simulink model "Pointmass_eom_v1_0_R2018B"  (R2018b)
settings: Solver=ode4  StartTime=0.0  StopTime=simInit.TSIM  FixedStep=simInit.dt  MaxStep=simInit.dt  RelTol=1e-3
InitFcn:
  | close all
undefined symbols (not defined in the file or in its folder): base_windspeed, constr, DE2019, DiscIntNeverNeededParam, ENVMT, Lbooth, loiterStates, params, simInit, T
libraries: simulink x26, simulink_extras x2, aerolibconvert2 x1, aerolibwind2 x1
(part 1 of 4)
Description:
  | % Copyright 2020 Delft University of Technology
  | %
  | % Licensed under the Apache License, Version 2.0 (the "License");
  | % you may not use this file except in compliance with the License.
  | % You may obtain a copy of the License at
  | %
  | %      http://www.apache.org/licenses/LICENSE-2.0
  | %
  | % Unless required by applicable law or agreed to in writing, software
  | % distributed under the License is distributed on an "AS IS" BASIS,
  | % WITHOUT WARRANTIES OR CONDITIONS OF ANY KIND, either express or implied.
  | % See the License for the specific language governing permissions and
  | % limitations under the License.
settings Model: SimulationMode=accelerator  ExtModeTrigDuration=100  Creator=Sebastian  LastModifiedBy=dylaneijkelhof
settings SolverCC: SolverJacobianMethodControl=FullAnalytical
settings DataIOCC: SaveFormat=Structure  SignalLogging=off  DSMLogging=off  SaveTime=off  StateSaveName=tmp_raccel_xout  SignalLoggingName=logged_signals  LoggingFileName=log
settings OptimizationCC: EfficientMapNaN2IntZero=off  LifeSpan=inf
settings DebuggingCC: ArtificialAlgebraicLoopMsg=none  SaveWithDisabledLinksMsg=none  SaveWithParameterizedLinksMsg=none  MaskedZcDiagnostic=none  IgnoredZcDiagnostic=none  InheritedTsInSrcMsg=none  TasksWithSamePriorityMsg=none  SigSpecEnsureSampleTimeMsg=none  ParameterPrecisionLossMsg=none  UnconnectedInputMsg=none  UnconnectedOutputMsg=none  UnconnectedLineMsg=none  BusObjectLabelMismatch=none  RootOutportRequireBusObject=none  UnknownTsInhSupMsg=none  ModelReferenceDataLoggingMessage=none  ModelReferenceSymbolNameMessage=none  InitInArrayFormatMsg=none  SFUnusedDataAndEventsDiag=none  SFUnexpectedBacktrackingDiag=none  SFInvalidInputDataAccessInChartInitDiag=none  SFNoUnconditionalDefaultTransitionDiag=none  SFTransitionOutsideNaturalParentDiag=none  SFUnreachableExecutionPathDiag=none  SFUndirectedBroadcastEventsDiag=none  SFTransitionActionBeforeConditionDiag=none  SFTemporalDelaySmallerThanSampleTimeDiag=none  SFSelfTransitionDiag=none  SFExecutionAtInitializationDiag=none  SFMachineParentedDataDiag=none  UnitsInconsistencyMsg=none
settings HardwareCC: TargetBitPerLong=64  TargetBitPerPointer=64  TargetBitPerSizeT=64  TargetBitPerPtrDiffT=64  TargetLongLongMode=on  TargetIntDivRoundTo=Zero  TargetEndianess=LittleEndian  TargetWordSize=64  TargetHWDeviceType=MATLAB Host  ProdEqTarget=off
settings ModelReferenceCC: PropagateSignalLabelsOutOfModel=off
settings SFSimCC: SimUseLocalCustomCode=off
settings CodeAppCC: MaxIdLength=128
settings GRTTargetCC: TargetLangStandard=C89/C90 (ANSI)  CombineOutputUpdateFcns=off  GRTInterface=on
settings ConfigComp: CovMetricSettings=dw  CovHtmlReporting=on  CovSaveCumulativeToWorkspaceVar=on  CovSaveSingleToWorkspaceVar=on  CovExternalEMLEnable=off
settings SimscapeCC: SimscapeNormalizeSystem=off
settings ConfigurationSet: Description=SimMechanics 2G

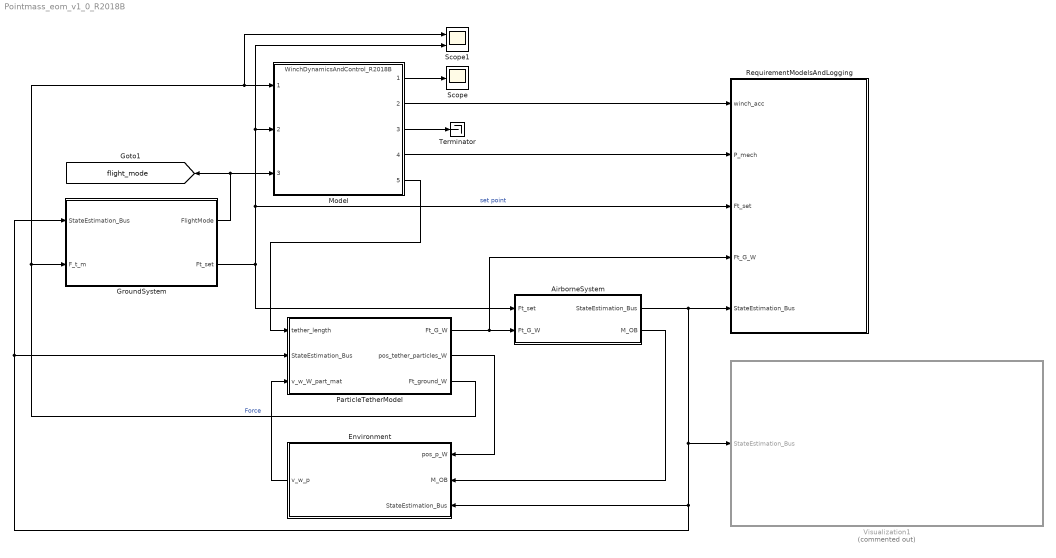
== system Pointmass_eom_v1_0_R2018B ==
  AirborneSystem : Subsystem
  Environment : Subsystem
  GroundSystem : Subsystem
  Model : ModelReference  ModelNameDialog=WinchDynamicsAndControl_R2018B.slx  ModelReferenceVersion=1.22542
  ParticleTetherModel : Subsystem
  RequirementModelsAndLogging : Subsystem  mask{log_sample_time=0.2}
  Scope : Scope
  Scope1 : Scope  NumInputPorts=2
  Terminator : Terminator
  Visualization1 : Subsystem  Commented=on  mask{sample_time_vis=1}
      mask prompts: sample_time_vis "sampletime"
      mask Display: image('DE2019_Aircraft.jpeg')
  tag scope: flight_mode=global
  wires:
  GroundSystem/1(FlightMode) -> Model/3, [flight_mode]
  GroundSystem/2(Ft_set) -> Scope1/2, Model/2, RequirementModelsAndLogging/3(Ft_set), AirborneSystem/1(Ft_set)  "set point"
  AirborneSystem/2(M_OB) -> Environment/2(M_OB)
  ParticleTetherModel/1(Ft_G_W) -> AirborneSystem/2(Ft_G_W), RequirementModelsAndLogging/4(Ft_G_W)
  AirborneSystem/1(StateEstimation_Bus) -> GroundSystem/1(StateEstimation_Bus), ParticleTetherModel/2(StateEstimation_Bus), Environment/3(StateEstimation_Bus), Visualization1/1(StateEstimation_Bus), RequirementModelsAndLogging/5(StateEstimation_Bus)
  ParticleTetherModel/2(pos_tether_particles_W) -> Environment/1(pos_p_W)
  Environment/1(v_w_p) -> ParticleTetherModel/3(v_w_W_part_mat)
  Model/1 -> Scope/1
  ParticleTetherModel/3(Ft_ground_W) -> Scope1/1, Model/1, GroundSystem/2(F_t_m)  "Force"
  Model/3 -> Terminator/1
  Model/2 -> RequirementModelsAndLogging/1(winch_acc)
  Model/4 -> RequirementModelsAndLogging/2(P_mech)
  Model/5 -> ParticleTetherModel/1(tether_length)

== system Pointmass_eom_v1_0_R2018B/AirborneSystem ==
  Ft_set : Inport
  Ft_G_W : Inport  Port=2
  AeroAndPropForces1 : Subsystem
  AttitudeDynamics : Subsystem
  Bus Selector : BusSelector  OutputSignals=airdata
  Delay2 : Delay  DelayLength=1  InitialCondition=[0;0;DE2019.mass*ENVMT.g]
  Dot Product : DotProduct  InputSameDT=on  OutDataTypeStr=Inherit: Inherit via internal rule
  FlightControlSystem : Subsystem
  PointMassEOM : Subsystem
  Sqrt : Sqrt  SaturateOnIntegerOverflow=on
  alpha : Scope  NumInputPorts=2
  mu : Scope  NumInputPorts=2
  StateEstimation_Bus : Outport  VectorParamsAs1DForOutWhenUnconnected=off
  M_OB : Outport  Port=2  VectorParamsAs1DForOutWhenUnconnected=off
  wires:
  PointMassEOM/2(StateEstimation_Bus) -> StateEstimation_Bus/1, FlightControlSystem/4(StateEstimation_Bus), Bus Selector/1  "StateEstimation_Bus"
  PointMassEOM/1(M_OB) -> M_OB/1
  Ft_G_W/1 -> PointMassEOM/1(F_t_W), Dot Product/1, Dot Product/2
  Dot Product/1 -> Sqrt/1
  Ft_set/1 -> FlightControlSystem/1(Ft_set)  "Ft_set"
  Sqrt/1 -> FlightControlSystem/2(Ft_tot)  "Ft_tot"
  FlightControlSystem/3(beta_c) -> PointMassEOM/4(beta_c)
  Delay2/1 -> FlightControlSystem/3(F_a_B_hat)
  AeroAndPropForces1/2(F_a_B) -> Delay2/1, PointMassEOM/6(F_a_B)  "Aero"
  FlightControlSystem/4(throttle) -> AeroAndPropForces1/1(throttle)  "throttle"
  Bus Selector/1 -> AeroAndPropForces1/2(air_data)  "<airdata>"
  AeroAndPropForces1/1(F_p_B) -> PointMassEOM/5(F_p_B)  "Propulsion"
  FlightControlSystem/1(mu_a_cmd) -> mu/1, AttitudeDynamics/1(mu_a_cmd)
  FlightControlSystem/2(alpha_a_cmd) -> alpha/1, AttitudeDynamics/2(alpha_a_cmd)
  AttitudeDynamics/1(mu_a) -> mu/2, PointMassEOM/2(mu_a_c)
  AttitudeDynamics/2(alpha_a) -> PointMassEOM/3(alpha_c), alpha/2

== system Pointmass_eom_v1_0_R2018B/Environment ==
  pos_p_W : Inport
  M_OB : Inport  Port=2
  StateEstimation_Bus : Inport  Port=3
  Bus Selector : BusSelector  OutputSignals=pos_G_O_m
  Constant4 : Constant  Value=ENVMT.windDirection_rad
  Delay : Delay  DelayLength=1  InitialCondition=zeros(3,1)
  Gain : Gain  Gain=-1
  Gain1 : Gain  Gain=-1
  MATLAB Function : MATLAB Function  TreatAsAtomicUnit=on
  Product : Product  Multiplication=Matrix(*)
  Reshape1 : Reshape  OutputDimensionality=Column vector (2-D)
  Selector : Selector  InputPortWidth=3  IndexOptions=Index vector (dialog)  Indices=3  OutputSizes=1
  Selector3 : Selector  InputPortWidth=3*T.np  IndexOptions=Index vector (dialog)  Indices=3:3:3*T.np  OutputSizes=1
  ShearWind : Subsystem  mask{Wdeg=ENVMT.windDirection_rad*180/pi}
      mask prompts: Wdeg "Windirection"
  Windshear : Subsystem
  v_w_p : Outport  VectorParamsAs1DForOutWhenUnconnected=off
  tag scope: vel_W_W=global
  wires:
  Bus Selector/1 -> Selector/1  "<pos_G_O_m>"
  Selector/1 -> Gain/1
  MATLAB Function/1(vec_W) -> Reshape1/1
  StateEstimation_Bus/1 -> Bus Selector/1
  Product/1 -> MATLAB Function/1(vec_O)
  M_OB/1 -> Product/1, Windshear/1(DCM)
  Windshear/1(V_shear_mDs) -> Gain1/1
  Gain1/1 -> Product/2
  Gain/1 -> Windshear/2(altitude)
  Constant4/1 -> MATLAB Function/2(wind_direction_rad)
  Reshape1/1 -> Delay/1
  Selector3/1 -> ShearWind/1(Altitude_p_vec)
  pos_p_W/1 -> Selector3/1
  ShearWind/1(v_w_p) -> v_w_p/1
  Delay/1 -> [vel_W_W]

== system Pointmass_eom_v1_0_R2018B/GroundSystem ==
  StateEstimation_Bus : Inport
  F_t_m : Inport  Port=2
  Bus Selector : BusSelector  OutputSignals=pos_G_W,airdata,longlat
  Demux : Demux  Outputs=2
  GroundControl : Subsystem
  Selector : Selector  InputPortWidth=3  IndexOptions=Index vector (dialog)  Indices=1  OutputSizes=1
  Selector1 : Selector  InputPortWidth=3  IndexOptions=Index vector (dialog)  Indices=1  OutputSizes=1
  Selector3 : Selector  InputPortWidth=2  IndexOptions=Index vector (dialog)  Indices=1  OutputSizes=1
  StateMachine : Subsystem
  FlightMode : Outport  VectorParamsAs1DForOutWhenUnconnected=off
  Ft_set : Outport  Port=2  VectorParamsAs1DForOutWhenUnconnected=off
  tag scope: phi0_update=global
  wires:
  Selector/1 -> StateMachine/2(Va)
  Bus Selector/2 -> Selector/1  "<airdata>"
  Bus Selector/1 -> StateMachine/1(pos_W)  "<pos_G_W>"
  StateEstimation_Bus/1 -> Bus Selector/1
  Demux/1 -> StateMachine/3(longitude)
  StateMachine/2(Ft_set) -> Ft_set/1
  Demux/2 -> StateMachine/4(lattitude)
  [cross_track_error] -> StateMachine/6(cross_track_error)
  F_t_m/1 -> StateMachine/7(F_t_m)
  Bus Selector/3 -> Selector3/1, Demux/1  "<longlat>"
  StateMachine/1(FlightMode) -> GroundControl/1(flightMode), FlightMode/1
  Selector1/1 -> [phi0_update]
  GroundControl/1(path_update) -> Selector1/1, StateMachine/5(path_update)
  Selector3/1 -> GroundControl/2(long)
  GroundControl/2(lat_init) -> StateMachine/8(lat_init)

== system Pointmass_eom_v1_0_R2018B/ParticleTetherModel ==
  tether_length : Inport
  StateEstimation_Bus : Inport  Port=2
  v_w_W_part_mat : Inport  Port=3
  Bus Selector : BusSelector  OutputSignals=pos_G_W,vel_W
  Delay : Delay  DelayLength=1  InitialCondition=zeros(3,1)
  Delay1 : Delay  DelayLength=1  InitialCondition=zeros(3,1)
  Dot Product : DotProduct  InputSameDT=on  OutDataTypeStr=Inherit: Inherit via internal rule
  Dot Product1 : DotProduct  Commented=on  InputSameDT=on  OutDataTypeStr=Inherit: Inherit via internal rule
  Gain : Gain  Gain=-1
  Integrator : Integrator  InitialCondition=simInit.vel_p_init
  Integrator1 : Integrator  InitialCondition=simInit.pos_p_init
  Scope : Scope  Commented=on  NumInputPorts=2
  Selector1 : Selector  InputPortWidth=3*T.np  IndexOptions=Index vector (dialog)  Indices=3:3:3*T.np  OutputSizes=1
  Selector2 : Selector  InputPortWidth=3*T.np  IndexOptions=Index vector (dialog)  Indices=2:3:3*T.np-1  OutputSizes=1
  Selector3 : Selector  InputPortWidth=3*T.np  IndexOptions=Index vector (dialog)  Indices=1:3:3*T.np-2  OutputSizes=1
  Sqrt : Sqrt  SaturateOnIntegerOverflow=on
  Sqrt1 : Sqrt  Commented=on  SaturateOnIntegerOverflow=on
  Tethermodel : ModelReference  ModelNameDialog=Tethermodel_R2018B.slx  ModelReferenceVersion=1.22531
  Ft_G_W : Outport  VectorParamsAs1DForOutWhenUnconnected=off
  pos_tether_particles_W : Outport  Port=2  VectorParamsAs1DForOutWhenUnconnected=off
  Ft_ground_W : Outport  Port=3  VectorParamsAs1DForOutWhenUnconnected=off
  tag scope: p_t_x=global, p_t_y=global, p_t_z=global
  wires:
  Tethermodel/2 -> Delay/1
  Tethermodel/3 -> Gain/1
  Gain/1 -> Delay1/1
  v_w_W_part_mat/1 -> Tethermodel/6
  Integrator/1 -> Integrator1/1, Tethermodel/1
  Tethermodel/1 -> Integrator/1
  Delay/1 -> Dot Product/2, Dot Product/1
  StateEstimation_Bus/1 -> Bus Selector/1
  Bus Selector/1 -> Tethermodel/4  "<pos_G_W>"
  Bus Selector/2 -> Tethermodel/5  "<vel_W>"
  Selector3/1 -> [p_t_x]
  Selector1/1 -> [p_t_z]
  Selector2/1 -> [p_t_y]
  Integrator1/1 -> Tethermodel/2, Selector3/1, Selector2/1, Selector1/1, pos_tether_particles_W/1
  Dot Product/1 -> Sqrt/1
  Sqrt/1 -> Ft_ground_W/1, Scope/1
  Dot Product1/1 -> Sqrt1/1
  Sqrt1/1 -> Scope/2
  Delay1/1 -> Dot Product1/1, Dot Product1/2, Ft_G_W/1
  tether_length/1 -> Tethermodel/3

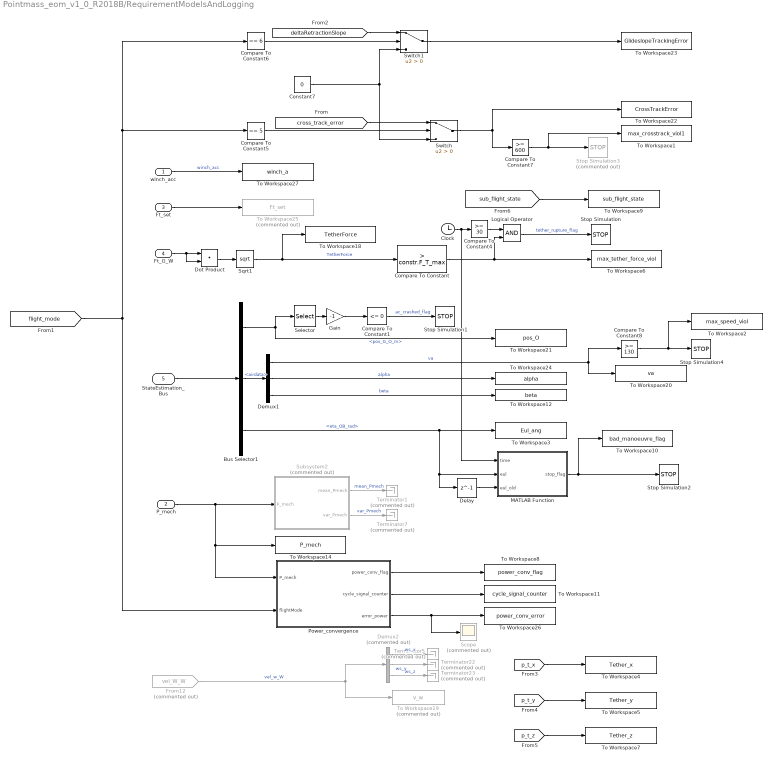
== system Pointmass_eom_v1_0_R2018B/RequirementModelsAndLogging ==
  winch_acc : Inport
  P_mech : Inport  Port=2
  Ft_set : Inport  Port=3
  Ft_G_W : Inport  Port=4
  StateEstimation_Bus : Inport  Port=5
  Bus Selector1 : BusSelector  OutputSignals=pos_G_O_m,airdata,eta_OB_rad
  Clock : Clock
  Compare To Constant : simulink/Logic and Bit Operations/Compare To Constant  relop=>  const=constr.F_T_max  OutDataTypeStr=boolean
  Compare To Constant1 : simulink/Logic and Bit Operations/Compare To Constant  relop=<=  const=0  OutDataTypeStr=boolean
  Compare To Constant4 : simulink/Logic and Bit Operations/Compare To Constant  relop=>=  const=30  OutDataTypeStr=boolean
  Compare To Constant5 : simulink/Logic and Bit Operations/Compare To Constant  relop===  const=5  OutDataTypeStr=boolean
  Compare To Constant6 : simulink/Logic and Bit Operations/Compare To Constant  relop===  const=6  OutDataTypeStr=boolean
  Compare To Constant7 : simulink/Logic and Bit Operations/Compare To Constant  relop=>=  const=600  OutDataTypeStr=boolean
  Compare To Constant8 : simulink/Logic and Bit Operations/Compare To Constant  relop=>=  const=130  OutDataTypeStr=boolean
  Constant7 : Constant  Value=0
  Delay : Delay  DelayLength=1  InitialCondition=zeros(3,1)
  Demux1 : Demux  Outputs=3
  Demux2 : Demux  Commented=on  Outputs=3
  Dot Product : DotProduct  InputSameDT=on  OutDataTypeStr=Inherit: Inherit via internal rule
  From12 : From  Commented=on  GotoTag=vel_W_W  TagVisibility=global
  Gain : Gain  Gain=-1
  Logical Operator : Logic  AllPortsSameDT=off  OutDataTypeStr=boolean
  MATLAB Function : MATLAB Function  TreatAsAtomicUnit=on
  Power_convergence : Subsystem  mask{sample_time=simInit.Ts_power_conv_check, threshold=130000}
  Scope : Scope  Commented=on
  Selector : Selector  InputPortWidth=3  IndexOptions=Index vector (dialog)  Indices=3  OutputSizes=1
  Sqrt1 : Sqrt  SaturateOnIntegerOverflow=on
  Stop Simulation{,1..2,4} (4 alike) : Stop
  Stop Simulation3 : Stop  Commented=on
  Subsystem2 : Subsystem  Commented=on
  Switch : Switch  Criteria=u2 > Threshold
  Switch1 : Switch  Criteria=u2 > Threshold
  Terminator{1,5,7,22..23} (5 alike) : Terminator  Commented=on
  To Workspace1 : ToWorkspace  VariableName=max_crosstrack_viol1  SampleTime=-1
      settings: MaxDataPoints=1
  To Workspace10 : ToWorkspace  VariableName=bad_manoeuvre_flag  SampleTime=-1
      settings: MaxDataPoints=1
  To Workspace11 : ToWorkspace  VariableName=cycle_signal_counter  SaveFormat=Timeseries  SampleTime=-1
      settings: MaxDataPoints=1  Save2DSignal=2-D array (concatenate along first dimension)
  To Workspace12 : ToWorkspace  VariableName=beta  SaveFormat=Timeseries  SampleTime=simInit.AttLoggingTs
      settings: Save2DSignal=2-D array (concatenate along first dimension)
  To Workspace14 : ToWorkspace  VariableName=P_mech  SaveFormat=Timeseries  SampleTime=simInit.PLoggingTs
  To Workspace18 : ToWorkspace  VariableName=TetherForce  SaveFormat=Timeseries  SampleTime=simInit.FtLoggingTs
  To Workspace19 : ToWorkspace  Commented=on  VariableName=v_w  SaveFormat=Timeseries  SampleTime=simInit.vWLoggingTs
  To Workspace2 : ToWorkspace  VariableName=max_speed_viol  SampleTime=-1
      settings: MaxDataPoints=1
  To Workspace20 : ToWorkspace  VariableName=va  SaveFormat=Timeseries  SampleTime=simInit.PLoggingTs
      settings: Save2DSignal=2-D array (concatenate along first dimension)
  To Workspace21 : ToWorkspace  VariableName=pos_O  SaveFormat=Timeseries  SampleTime=simInit.PLoggingTs
      settings: Save2DSignal=2-D array (concatenate along first dimension)
  To Workspace22 : ToWorkspace  VariableName=CrossTrackError  SaveFormat=Timeseries  SampleTime=simInit.CteLoggingTs
      settings: Save2DSignal=2-D array (concatenate along first dimension)
  To Workspace23 : ToWorkspace  VariableName=GlideslopeTrackingError  SaveFormat=Timeseries  SampleTime=simInit.GSLoggingTs
      settings: Save2DSignal=2-D array (concatenate along first dimension)
  To Workspace24 : ToWorkspace  VariableName=alpha  SaveFormat=Timeseries  SampleTime=simInit.AttLoggingTs
      settings: Save2DSignal=2-D array (concatenate along first dimension)
  To Workspace25 : ToWorkspace  Commented=on  VariableName=Ft_set  SaveFormat=Timeseries  SampleTime=simInit.FtLoggingTs
  To Workspace26 : ToWorkspace  VariableName=power_conv_error  SaveFormat=Timeseries  SampleTime=-1
      settings: Save2DSignal=2-D array (concatenate along first dimension)
  To Workspace27 : ToWorkspace  VariableName=winch_a  SaveFormat=Timeseries  SampleTime=simInit.PLoggingTs
  To Workspace3 : ToWorkspace  VariableName=Eul_ang  SaveFormat=Timeseries  SampleTime=simInit.PLoggingTs
      settings: Save2DSignal=2-D array (concatenate along first dimension)
  To Workspace4 : ToWorkspace  VariableName=Tether_x  SaveFormat=Timeseries  SampleTime=simInit.PLoggingTs
      settings: Save2DSignal=2-D array (concatenate along first dimension)
  To Workspace5 : ToWorkspace  VariableName=Tether_y  SaveFormat=Timeseries  SampleTime=simInit.PLoggingTs
      settings: Save2DSignal=2-D array (concatenate along first dimension)
  To Workspace6 : ToWorkspace  VariableName=max_tether_force_viol  SampleTime=-1
      settings: MaxDataPoints=1
  To Workspace7 : ToWorkspace  VariableName=Tether_z  SaveFormat=Timeseries  SampleTime=simInit.PLoggingTs
      settings: Save2DSignal=2-D array (concatenate along first dimension)
  To Workspace8 : ToWorkspace  VariableName=power_conv_flag  SampleTime=-1
      settings: MaxDataPoints=1
  To Workspace9 : ToWorkspace  VariableName=sub_flight_state  SaveFormat=Timeseries  SampleTime=simInit.FtLoggingTs
  wires:
  Bus Selector1/1 -> Selector/1, To Workspace21/1  "<pos_G_O_m>"
  Gain/1 -> Compare To Constant1/1
  Compare To Constant1/1 -> Stop Simulation1/1  "ac_crashed_flag"
  Selector/1 -> Gain/1
  winch_acc/1 -> To Workspace27/1  "winch_acc"
  Logical Operator/1 -> Stop Simulation/1  "tether_rupture_flag"
  Sqrt1/1 -> To Workspace18/1, Compare To Constant/1  "TetherForce"
  StateEstimation_Bus/1 -> Bus Selector1/1
  Power_convergence/1(power_conv_flag) -> To Workspace8/1
  Power_convergence/2(cycle_signal_counter) -> To Workspace11/1
  From12/1 -> Demux2/1, To Workspace19/1  "vel_w_W"
  Bus Selector1/2 -> Demux1/1  "<airdata>"
  Switch/1 -> To Workspace22/1, Compare To Constant7/1
  Subsystem2/1(mean_Pmech) -> Terminator1/1  "mean_Pmech"
  Subsystem2/2(var_Pmech) -> Terminator7/1  "var_Pmech"
  Demux1/1 -> Compare To Constant8/1, To Workspace20/1  "va"
  Demux1/2 -> To Workspace24/1  "alpha"
  Demux1/3 -> To Workspace12/1  "beta"
  Demux2/3 -> Terminator23/1  "ws_z"
  Demux2/2 -> Terminator22/1  "ws_y"
  Demux2/1 -> Terminator5/1  "ws_x"
  Ft_G_W/1 -> Dot Product/2, Dot Product/1
  Dot Product/1 -> Sqrt1/1
  Clock/1 -> MATLAB Function/1(time), Compare To Constant4/1
  Compare To Constant4/1 -> Logical Operator/1
  Compare To Constant/1 -> Logical Operator/2, To Workspace6/1
  [flight_mode] -> Compare To Constant6/1, Compare To Constant5/1, Power_convergence/2(flightMode)
  P_mech/1 -> Power_convergence/1(P_mech), To Workspace14/1, Subsystem2/1(P_mech)
  Compare To Constant5/1 -> Switch/2
  [cross_track_error] -> Switch/1
  Switch1/1 -> To Workspace23/1
  [deltaRetractionSlope] -> Switch1/1
  Compare To Constant6/1 -> Switch1/2
  Constant7/1 -> Switch1/3, Switch/3
  Ft_set/1 -> To Workspace25/1
  Power_convergence/3(error_power) -> Scope/1, To Workspace26/1
  Compare To Constant7/1 -> Stop Simulation3/1, To Workspace1/1
  Compare To Constant8/1 -> To Workspace2/1, Stop Simulation4/1
  [p_t_y] -> To Workspace5/1
  [p_t_x] -> To Workspace4/1
  [p_t_z] -> To Workspace7/1
  [sub_flight_state] -> To Workspace9/1
  Bus Selector1/3 -> To Workspace3/1, Delay/1, MATLAB Function/2(eul)  "<eta_OB_rad>"
  Delay/1 -> MATLAB Function/3(eul_old)
  MATLAB Function/1(stop_flag) -> Stop Simulation2/1, To Workspace10/1

== system Pointmass_eom_v1_0_R2018B/Visualization1 ==
  StateEstimation_Bus : Inport
  Bus Selector : BusSelector  OutputSignals=pos_G_O_m,eta_OB_rad
  Clock2 : Clock
  Constant : Constant  Value=ENVMT.windDirection_rad
  Constant1 : Constant  Value=params.a_booth
  Constant2 : Constant  Value=params.b_booth
  Constant3 : Constant  Value=T.np
  Mux : Mux  Inputs=9
  Mux1 : Mux  Inputs=3
  Rate Transition1 : RateTransition  OutPortSampleTime=sample_time_vis
  Rate Transition2 : RateTransition  InitialCondition=simInit.pos_O_init  OutPortSampleTime=sample_time_vis
  Rate Transition3 : RateTransition  InitialCondition=zeros(3,1)  OutPortSampleTime=sample_time_vis
  Rate Transition4 : RateTransition  OutPortSampleTime=sample_time_vis
  Rate Transition5 : RateTransition  InitialCondition=simInit.pos_p_init(1:3:3*T.np-2)  OutPortSampleTime=sample_time_vis
  Rate Transition6 : RateTransition  OutPortSampleTime=sample_time_vis
  Rate Transition7 : RateTransition  InitialCondition=simInit.pos_p_init(2:3:3*T.np-1)  OutPortSampleTime=sample_time_vis
  Rate Transition8 : RateTransition  InitialCondition=simInit.pos_p_init(3:3:3*T.np)  OutPortSampleTime=sample_time_vis
  Rate Transition9 : RateTransition  InitialCondition=[params.a_booth;params.b_booth;params.phi0_booth]  OutPortSampleTime=sample_time_vis
  To Workspace : ToWorkspace  Commented=on  VariableName=save_visualization  SaveFormat=Timeseries  SampleTime=-1
  advanced_graphical_model : MATLABFcn  MATLABFcn=drawVehicle_v3st_twin  OutputDimensions=0
  wires:
  Bus Selector/2 -> Rate Transition3/1  "<eta_OB_rad>"
  Bus Selector/1 -> Rate Transition2/1  "<pos_G_O_m>"
  StateEstimation_Bus/1 -> Bus Selector/1
  Rate Transition3/1 -> Mux/2
  Rate Transition2/1 -> Mux/1
  Constant3/1 -> Rate Transition6/1
  Rate Transition6/1 -> Mux/4
  Mux/1 -> advanced_graphical_model/1, To Workspace/1  "visualization_stuff"
  Clock2/1 -> Rate Transition1/1
  Rate Transition1/1 -> Mux/3
  Rate Transition4/1 -> Mux/5
  Constant/1 -> Rate Transition4/1
  [p_t_z] -> Rate Transition8/1
  [p_t_y] -> Rate Transition7/1
  [p_t_x] -> Rate Transition5/1
  Rate Transition5/1 -> Mux/7
  Rate Transition7/1 -> Mux/8
  Rate Transition8/1 -> Mux/9
  Mux1/1 -> Rate Transition9/1
  Rate Transition9/1 -> Mux/6
  Constant1/1 -> Mux1/1
  Constant2/1 -> Mux1/2
  [phi0_update] -> Mux1/3

== system Pointmass_eom_v1_0_R2018B/AirborneSystem/AeroAndPropForces1 ==
  throttle : Inport
  air_data : Inport  Port=2
  1-D Lookup Table : Lookup_n-D  NumberOfTableDimensions=1  BreakpointsForDimension1=DE2019.initAircraft.alpha  BreakpointsForDimension2=[1 1]  Table=DE2019.initAircraft.wing_cL_Static'  InternalRulePriority=Speed  RndMeth=Simplest  InputSameDT=on
  1-D Lookup Table1 : Lookup_n-D  NumberOfTableDimensions=1  BreakpointsForDimension1=DE2019.initAircraft.alpha  BreakpointsForDimension2=[1 1]  Table=DE2019.initAircraft.wing_cD_Static'  InternalRulePriority=Speed  RndMeth=Simplest  InputSameDT=on
  1-D Lookup Table2 : Lookup_n-D  NumberOfTableDimensions=1  BreakpointsForDimension1=DE2019.alpha  BreakpointsForDimension2=[1 1]  Table=DE2019.el_cL'  InternalRulePriority=Speed  RndMeth=Simplest  InputSameDT=on
  1-D Lookup Table3 : Lookup_n-D  NumberOfTableDimensions=1  BreakpointsForDimension1=DE2019.alpha  BreakpointsForDimension2=[1 1]  Table=DE2019.el_cD'  InternalRulePriority=Speed  RndMeth=Simplest  InputSameDT=on
  1-D Lookup Table4 : Lookup_n-D  NumberOfTableDimensions=1  BreakpointsForDimension1=DE2019.alpha  BreakpointsForDimension2=[1 1]  Table=DE2019.vs_cL'  InternalRulePriority=Speed  RndMeth=Simplest  InputSameDT=on
  1-D Lookup Table5 : Lookup_n-D  NumberOfTableDimensions=1  BreakpointsForDimension1=DE2019.alpha  BreakpointsForDimension2=[1 1]  Table=DE2019.vs_cD'  InternalRulePriority=Speed  RndMeth=Simplest  InputSameDT=on
  Aero_prop : MATLAB Function  TreatAsAtomicUnit=on
  Radians to Degrees : simulink_extras/Transformations/Radians to Degrees
  Radians to Degrees1 : simulink_extras/Transformations/Radians to Degrees
  Saturation : Saturate  UpperLimit=max(DE2019.initAircraft.alpha)  LowerLimit=min(DE2019.initAircraft.alpha)
  Saturation1 : Saturate  UpperLimit=max(DE2019.alpha)  LowerLimit=min(DE2019.alpha)
  Saturation2 : Saturate  UpperLimit=max(DE2019.alpha)  LowerLimit=min(DE2019.alpha)
  Scope : Scope  Commented=on
  Selector : Selector  Commented=on  InputPortWidth=3  IndexOptions=Index vector (dialog)  Indices=[1]  OutputSizes=1
  Selector1 : Selector  Commented=on  InputPortWidth=3  IndexOptions=Index vector (dialog)  Indices=2  OutputSizes=1
  Selector2 : Selector  Commented=on  InputPortWidth=3  IndexOptions=Index vector (dialog)  Indices=3  OutputSizes=1
  Velocity : Scope  Commented=on
  alpha : Scope  Commented=on
  alpha select : Selector  InputPortWidth=3  IndexOptions=Index vector (dialog)  Indices=2  OutputSizes=1
  beta select : Selector  InputPortWidth=3  IndexOptions=Index vector (dialog)  Indices=3  OutputSizes=1
  F_p_B : Outport  VectorParamsAs1DForOutWhenUnconnected=off
  F_a_B : Outport  Port=2  VectorParamsAs1DForOutWhenUnconnected=off
  wires:
  Aero_prop/1(F_p_B) -> F_p_B/1
  throttle/1 -> Aero_prop/2(delta_t)
  Selector/1 -> Velocity/1
  Selector1/1 -> alpha/1
  1-D Lookup Table/1 -> Aero_prop/3(cl_w)
  1-D Lookup Table1/1 -> Aero_prop/4(cd_w)
  Saturation/1 -> 1-D Lookup Table/1, 1-D Lookup Table1/1
  Saturation1/1 -> 1-D Lookup Table3/1, 1-D Lookup Table2/1
  alpha select/1 -> Radians to Degrees/1
  Radians to Degrees/1 -> Saturation1/1, Saturation/1
  1-D Lookup Table2/1 -> Aero_prop/5(cl_e)
  1-D Lookup Table3/1 -> Aero_prop/6(cd_e)
  1-D Lookup Table4/1 -> Aero_prop/7(cl_r)
  1-D Lookup Table5/1 -> Aero_prop/8(cd_r)
  beta select/1 -> Radians to Degrees1/1
  Radians to Degrees1/1 -> Saturation2/1
  Saturation2/1 -> 1-D Lookup Table4/1, 1-D Lookup Table5/1
  Selector2/1 -> Scope/1
  Aero_prop/2(F_a_B) -> F_a_B/1, Selector2/1
  air_data/1 -> Selector/1, Selector1/1, Aero_prop/1(airdata), beta select/1, alpha select/1

== system Pointmass_eom_v1_0_R2018B/AirborneSystem/AttitudeDynamics ==
  mu_a_cmd : Inport
  alpha_a_cmd : Inport  Port=2
  Scope : Scope  Commented=on  NumInputPorts=2
  SecondOrderReferenceModel_alpha_a : Subsystem  mask{omega0_max=params.w0_alpha, omega0_min=0, dynP_max=1.5312e+03, dynP_min=245.0000, zeta0=0.7, y_max=constr.alpha_a_max, y_min=constr.alpha_a_min, yd_max=inf, yd_min=-inf, y2d_max=inf, y2d_min=-inf}
      mask prompts: dynP_max "max. dynamic pressure"; dynP_min "min. dynamic pressure"
  SecondOrderReferenceModel_mu_a : Subsystem  mask{omega0_max=params.w0_mu, omega0_min=0, dynP_max=1.5312e+03, dynP_min=245.0000, zeta0=1, y_max=constr.mu_a_max, y_min=-constr.mu_a_max, yd_max=inf, yd_min=-inf, y2d_max=inf, y2d_min=-inf}
      mask prompts: dynP_max "max. dynamic pressure"; dynP_min "min. dynamic pressure"
  mu_a : Outport  VectorParamsAs1DForOutWhenUnconnected=off
  alpha_a : Outport  Port=2  VectorParamsAs1DForOutWhenUnconnected=off
  wires:
  mu_a_cmd/1 -> SecondOrderReferenceModel_mu_a/1(y_cmd)
  SecondOrderReferenceModel_alpha_a/1(y_ref) -> Scope/1, alpha_a/1  "alpha_a"
  alpha_a_cmd/1 -> Scope/2, SecondOrderReferenceModel_alpha_a/1(y_cmd)
  SecondOrderReferenceModel_mu_a/1(y_ref) -> mu_a/1  "mu_a"

== system Pointmass_eom_v1_0_R2018B/AirborneSystem/FlightControlSystem ==
  Ft_set : Inport
  Ft_tot : Inport  Port=2
  F_a_B_hat : Inport  Port=3
  StateEstimation_Bus : Inport  Port=4
  AirspeedController : Subsystem
  Bus Selector : BusSelector  OutputSignals=airdata,pathangles_a
  Constant : Constant  Value=0
  PathFollowingController : Subsystem
  Rate Transition : RateTransition  OutPortSampleTime=0.001
  Rate Transition1 : RateTransition  OutPortSampleTime=0.001
  Selector : Selector  InputPortWidth=3  IndexOptions=Index vector (dialog)  Indices=1  OutputSizes=1
  Selector1 : Selector  InputPortWidth=3  IndexOptions=Index vector (dialog)  Indices=2  OutputSizes=1
  Selector2 : Selector  InputPortWidth=2  IndexOptions=Index vector (dialog)  Indices=2  OutputSizes=1
  mu_a_cmd : Outport  VectorParamsAs1DForOutWhenUnconnected=off
  alpha_a_cmd : Outport  Port=2  VectorParamsAs1DForOutWhenUnconnected=off
  beta_c : Outport  Port=3  VectorParamsAs1DForOutWhenUnconnected=off
  throttle : Outport  Port=4  VectorParamsAs1DForOutWhenUnconnected=off
  wires:
  StateEstimation_Bus/1 -> PathFollowingController/4(StateEstimation_Bus), Bus Selector/1
  Ft_set/1 -> PathFollowingController/1(ft_set)
  Ft_tot/1 -> PathFollowingController/2(f_t_m), AirspeedController/5(Ft_set)
  Bus Selector/1 -> Selector/1, Selector1/1  "<airdata>"
  Selector2/1 -> AirspeedController/3(gamma_a)
  Selector/1 -> AirspeedController/1(Va)
  Selector1/1 -> AirspeedController/2(alpha)
  F_a_B_hat/1 -> AirspeedController/4(F_a_B), PathFollowingController/3(F_a_B_est)
  Bus Selector/2 -> Selector2/1  "<pathangles_a>"
  AirspeedController/1(Thrust_force) -> throttle/1
  Constant/1 -> beta_c/1
  PathFollowingController/1(mu_a_cmd) -> Rate Transition/1
  PathFollowingController/2(alpha_a_cmd) -> Rate Transition1/1
  Rate Transition/1 -> mu_a_cmd/1
  Rate Transition1/1 -> alpha_a_cmd/1

== system Pointmass_eom_v1_0_R2018B/AirborneSystem/PointMassEOM ==
  F_t_W : Inport  PortDimensions=[3,1]
  mu_a_c : Inport  Port=2
  alpha_c : Inport  Port=3
  beta_c : Inport  Port=4
  F_p_B : Inport  Port=5  PortDimensions=[3,1]
  F_a_B : Inport  Port=6  PortDimensions=[3,1]
  Bus Creator1 : BusCreator  Inputs=13
  Constant : Constant  Value=0
  MATLAB Function3 : MATLAB Function  TreatAsAtomicUnit=on
  PointMassDynamics : Subsystem
  M_OB : Outport  PortDimensions=[3,3]  VectorParamsAs1DForOutWhenUnconnected=off
  StateEstimation_Bus : Outport  Port=2  VectorParamsAs1DForOutWhenUnconnected=off
  wires:
  mu_a_c/1 -> PointMassDynamics/1(mu_a_c), Bus Creator1/1  "mu_a"
  PointMassDynamics/11(M_OB) -> M_OB/1
  PointMassDynamics/5(pathangles_a) -> Bus Creator1/6  "pathangles_a"
  PointMassDynamics/4(pathangles_k) -> Bus Creator1/5  "pathangles_k"
  PointMassDynamics/6(eta_EULER) -> Bus Creator1/7  "eta_OB_rad"
  PointMassDynamics/7(longlat) -> Bus Creator1/8  "longlat"
  PointMassDynamics/3(vel_k_O) -> Bus Creator1/4  "vel_K_O_mDs"
  Bus Creator1/1 -> StateEstimation_Bus/1
  PointMassDynamics/2(pos_O) -> Bus Creator1/3  "pos_G_O_m"
  MATLAB Function3/1(v_w_O) -> PointMassDynamics/7(v_w_O), Bus Creator1/13  "v_w_hat_O"
  [vel_W_W] -> MATLAB Function3/1(v_w_W)
  PointMassDynamics/9(pos_W) -> Bus Creator1/10  "pos_G_W"
  PointMassDynamics/10(v_k_W) -> Bus Creator1/11  "vel_W"
  PointMassDynamics/1(airdata) -> Bus Creator1/2  "airdata"
  PointMassDynamics/8(vel_k_B) -> Bus Creator1/9  "v_k_B"
  F_p_B/1 -> PointMassDynamics/5(F_p_B)
  F_t_W/1 -> PointMassDynamics/6(F_t_W)
  F_a_B/1 -> PointMassDynamics/4(F_a_B)
  alpha_c/1 -> PointMassDynamics/2(alpha_c)  "alpha"
  beta_c/1 -> PointMassDynamics/3(beta_c)  "beta"
  Constant/1 -> Bus Creator1/12  "a_tot"

== system Pointmass_eom_v1_0_R2018B/Environment/ShearWind ==
  Altitude_p_vec : Inport  OutDataTypeStr=double  Unit=m
  3ft-->inf : Saturate  UpperLimit=inf  LowerLimit=3
  Length Conversion : aerolibconvert2/Length Conversion  IU=m  OU=ft
  MATLAB Function : MATLAB Function  TreatAsAtomicUnit=on
  Product : Product  Inputs=*/  InputSameDT=on  SaturateOnIntegerOverflow=on  OutDataTypeStr=Inherit: Same as first input
  Product1 : Product  InputSameDT=on  SaturateOnIntegerOverflow=on  OutDataTypeStr=Inherit: Same as first input
  Reshape : Reshape  OutputDimensionality=Column vector (2-D)
  Wdeg2 : Constant  Value=base_windspeed  OutDataTypeStr=Inherit: Inherit via back propagation
  h/z0 : Gain  Gain=1/0.15  SaturateOnIntegerOverflow=on  OutDataTypeStr=Inherit: Same as input  ParamDataTypeStr=Inherit: Same as input
  ln(h/z0) : Math  Operator=log  SaturateOnIntegerOverflow=on
  ln(ref_height/z0) : Math  Operator=log  SaturateOnIntegerOverflow=on
  ref_height/z0 [ft] : Constant  Value=20/0.15  OutDataTypeStr=Inherit: Inherit via back propagation
  v_w_p : Outport  Unit=m/s  VectorParamsAs1DForOutWhenUnconnected=off
  wires:
  3ft-->inf/1 -> h/z0/1
  Product/1 -> Product1/1
  Wdeg2/1 -> Product1/2
  ref_height/z0 [ft]/1 -> ln(ref_height/z0)/1
  h/z0/1 -> ln(h/z0)/1
  ln(ref_height/z0)/1 -> Product/2
  Reshape/1 -> MATLAB Function/1(v_w_u)
  ln(h/z0)/1 -> Product/1
  Product1/1 -> Reshape/1
  Length Conversion/1 -> 3ft-->inf/1
  MATLAB Function/1(v_w_p_mat) -> v_w_p/1
  Altitude_p_vec/1 -> Length Conversion/1

== system Pointmass_eom_v1_0_R2018B/Environment/Windshear ==
  DCM : Inport
  altitude : Inport  Port=2
  Math Function : Math  Operator=transpose  SaturateOnIntegerOverflow=on
  Wind Shear Model : aerolibwind2/Wind Shear Model  units=Metric (MKS)  phase=Category C - Terminal Flight Phase  W_20=base_windspeed  Wdeg=ENVMT.windDirection_rad*180/pi
  V_shear_mDs : Outport  VectorParamsAs1DForOutWhenUnconnected=off
  wires:
  altitude/1 -> Wind Shear Model/1
  DCM/1 -> Math Function/1
  Math Function/1 -> Wind Shear Model/2
  Wind Shear Model/1 -> V_shear_mDs/1

== system Pointmass_eom_v1_0_R2018B/GroundSystem/GroundControl ==
  flightMode : Inport
  long : Inport  Port=2
  Chart : Stateflow chart  TreatAsAtomicUnit=on
  Compare To Constant : simulink/Logic and Bit Operations/Compare To Constant  relop===  const=1  OutDataTypeStr=boolean
  Compare To Constant2 : simulink/Logic and Bit Operations/Compare To Constant  relop===  const=6  OutDataTypeStr=boolean
  Compare To Constant3 : simulink/Logic and Bit Operations/Compare To Constant  relop===  const=5  OutDataTypeStr=boolean
  Constant : Constant  Value=0
  Constant1 : Constant  Value=0
  Constant11 : Constant  Value=params.phi0_booth
  Constant9 : Constant  Value=params.transition_phi
  Gain4 : Gain  Gain=pi/180
  Gain7 : Gain  Gain=params.w0_decrease_init_phi0
  Integrator : Integrator  ExternalReset=rising  InitialConditionSource=external
  Logical Operator1 : Logic  Operator=OR  AllPortsSameDT=off  OutDataTypeStr=boolean
  Mux : Mux  Inputs=3
  Select_init_sol_for_pathfollowing : Stateflow chart  TreatAsAtomicUnit=on
  Sum3 : Sum  Inputs=|+-
  Switch : Switch  Criteria=u2 > Threshold
  Switch3 : Switch  Threshold=1
  initial_path_elevation : Constant  Value=params.initial_path_elevation
  path_update : Outport  PortDimensions=[3,1]  VectorParamsAs1DForOutWhenUnconnected=off
  lat_init : Outport  Port=2  VectorParamsAs1DForOutWhenUnconnected=off
  wires:
  Constant1/1 -> Mux/3
  Constant/1 -> Mux/2
  Mux/1 -> path_update/1
  Sum3/1 -> Gain7/1
  Select_init_sol_for_pathfollowing/1(sol_init) -> Gain4/1
  flightMode/1 -> Select_init_sol_for_pathfollowing/2(fm), Compare To Constant3/1, Compare To Constant2/1, Chart/2(fm)
  Compare To Constant2/1 -> Logical Operator1/2
  Switch/1 -> Sum3/1
  Compare To Constant3/1 -> Switch/2
  initial_path_elevation/1 -> Select_init_sol_for_pathfollowing/1(x)
  long/1 -> Chart/1(long)  "long"
  Chart/1(c_out) -> Switch3/2, Compare To Constant/1
  Gain4/1 -> Switch3/3, Integrator/3, lat_init/1, Switch/3
  Integrator/1 -> Sum3/2, Switch3/1
  Compare To Constant/1 -> Logical Operator1/1
  Logical Operator1/1 -> Integrator/2
  Gain7/1 -> Integrator/1
  Switch3/1 -> Mux/1
  Constant9/1 -> Select_init_sol_for_pathfollowing/3(transition_phi)
  Constant11/1 -> Switch/1

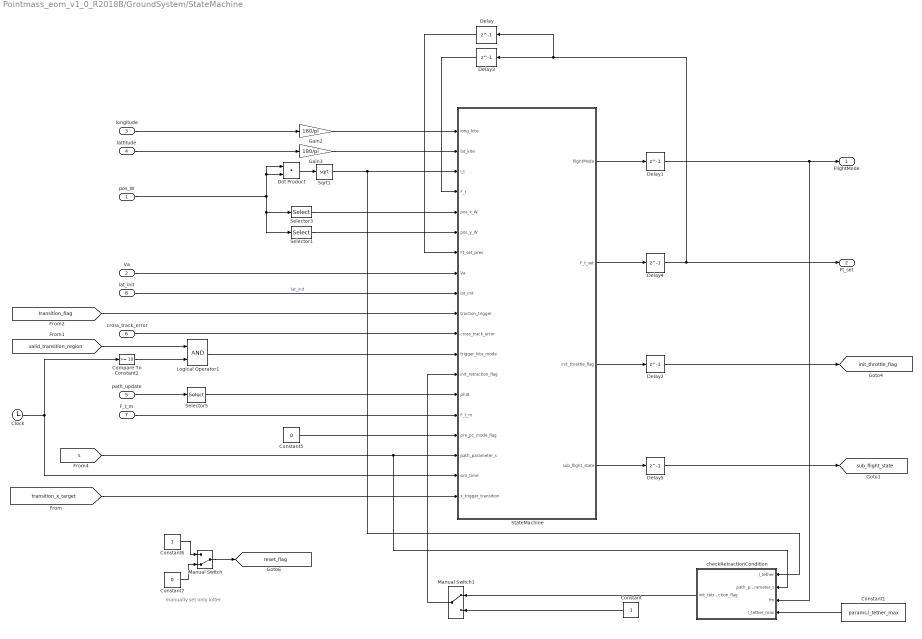
== system Pointmass_eom_v1_0_R2018B/GroundSystem/StateMachine ==
  note: manually set only loiter
  pos_W : Inport
  Va : Inport  Port=2
  longitude : Inport  Port=3
  lattitude : Inport  Port=4
  path_update : Inport  Port=5
  cross_track_error : Inport  Port=6
  F_t_m : Inport  Port=7
  lat_init : Inport  Port=8
  Clock : Clock
  Compare To Constant2 : simulink/Logic and Bit Operations/Compare To Constant  relop=>=  const=10  OutDataTypeStr=boolean
  Constant : Constant
  Constant1 : Constant  Value=params.l_tether_max
  Constant5 : Constant  Value=0
  Constant6 : Constant
  Constant7 : Constant  Value=0
  Delay : Delay  DelayLength=1  InitialCondition=100
  Delay1 : Delay  DelayLength=1
  Delay2 : Delay  DelayLength=1  InitialCondition=1
  Delay3 : Delay  DelayLength=1  InitialCondition=100
  Delay4 : Delay  DelayLength=1
  Delay5 : Delay  DelayLength=1  InitialCondition=1
  Dot Product : DotProduct  InputSameDT=on  OutDataTypeStr=Inherit: Inherit via internal rule
  Gain2 : Gain  Gain=180/pi
  Gain3 : Gain  Gain=180/pi
  Logical Operator1 : Logic  AllPortsSameDT=off  OutDataTypeStr=boolean
  Manual Switch : ManualSwitch  CurrentSetting=0
  Manual Switch1 : ManualSwitch
  Selector1 : Selector  InputPortWidth=3  IndexOptions=Index vector (dialog)  Indices=2  OutputSizes=1
  Selector3 : Selector  InputPortWidth=3  IndexOptions=Index vector (dialog)  Indices=1  OutputSizes=1
  Selector5 : Selector  InputPortWidth=3  IndexOptions=Index vector (dialog)  Indices=1  OutputSizes=1
  Sqrt1 : Sqrt  SaturateOnIntegerOverflow=on
  StateMachine : Stateflow chart  TreatAsAtomicUnit=on  mask{F_T_traction_set=params.F_t_traction_set, F_set_retraction=params.F_t_retraction_set, l_t_min=params.l_tether_min, l_t_max=params.l_tether_max, a_booth=params.a_booth, b_booth=params.b_booth, lat_trans=0, alpha1=params.ft_smooth_1, alpha2=params.ft_smooth_2, crosstrackerror_condition=params.crosstrackerror_condition, Vamin=constr.Va_min, Ft_set_loiter=loiterStates.Ft_set_loiter, alpha3=params.ft_smooth_3}
      mask prompts: F_T_traction_set "Traction force"; F_set_retraction "Retraction force"; l_t_min "Min. tether length"; l_t_max "Max. tether length"; a_booth "abooth"; b_booth "bbooth"; alpha1 "interpolation factor init kite (alpha1)"; alpha2 "interpolation factor retrac 2 trac"
  checkRetractionCondition : Stateflow chart  TreatAsAtomicUnit=on
  FlightMode : Outport  VectorParamsAs1DForOutWhenUnconnected=off
  Ft_set : Outport  Port=2  VectorParamsAs1DForOutWhenUnconnected=off
  tag scope: init_throttle_flag=global, reset_flag=global, sub_flight_state=global
  wires:
  Manual Switch1/1 -> StateMachine/13(init_retraction_flag)
  Constant1/1 -> checkRetractionCondition/4(l_tether_max)
  Va/1 -> StateMachine/8(Va)
  StateMachine/2(F_t_set) -> Delay4/1
  lattitude/1 -> Gain3/1
  longitude/1 -> Gain2/1
  Delay2/1 -> [init_throttle_flag]
  StateMachine/3(init_throttle_flag) -> Delay2/1
  Delay1/1 -> FlightMode/1, checkRetractionCondition/3(fm)
  [valid_transition_region] -> Logical Operator1/1
  Compare To Constant2/1 -> Logical Operator1/2
  Logical Operator1/1 -> StateMachine/12(trigger_kite_mode)
  cross_track_error/1 -> StateMachine/11(cross_track_error)
  Selector1/1 -> StateMachine/6(pos_y_W)
  Delay/1 -> StateMachine/7(Ft_set_prev)
  Dot Product/1 -> Sqrt1/1
  Selector3/1 -> StateMachine/5(pos_x_W)
  pos_W/1 -> Selector3/1, Selector1/1, Dot Product/1, Dot Product/2
  Gain2/1 -> StateMachine/1(long_kite)
  StateMachine/1(flightMode) -> Delay1/1
  Delay3/1 -> StateMachine/4(F_t)
  Selector5/1 -> StateMachine/14(phi0)
  path_update/1 -> Selector5/1
  Gain3/1 -> StateMachine/2(lat_kite)
  Sqrt1/1 -> checkRetractionCondition/1(l_tether), StateMachine/3(l_t)
  Delay4/1 -> Ft_set/1, Delay/1, Delay3/1
  StateMachine/4(sub_flight_state) -> Delay5/1
  F_t_m/1 -> StateMachine/15(F_t_m)
  Constant5/1 -> StateMachine/16(pre_pc_mode_flag)
  [transition_flag] -> StateMachine/10(traction_trigger)
  Constant6/1 -> Manual Switch/1
  Constant7/1 -> Manual Switch/2
  Manual Switch/1 -> [reset_flag]
  Clock/1 -> Compare To Constant2/1, StateMachine/18(sim_time)
  [s] -> checkRetractionCondition/2(path_parameter_s), StateMachine/17(path_parameter_s)
  lat_init/1 -> StateMachine/9(lat_init)  "lat_init"
  checkRetractionCondition/1(init_retraction_flag) -> Manual Switch1/1
  Constant/1 -> Manual Switch1/2
  Delay5/1 -> [sub_flight_state]
  [transition_x_target] -> StateMachine/19(x_trigger_transition)

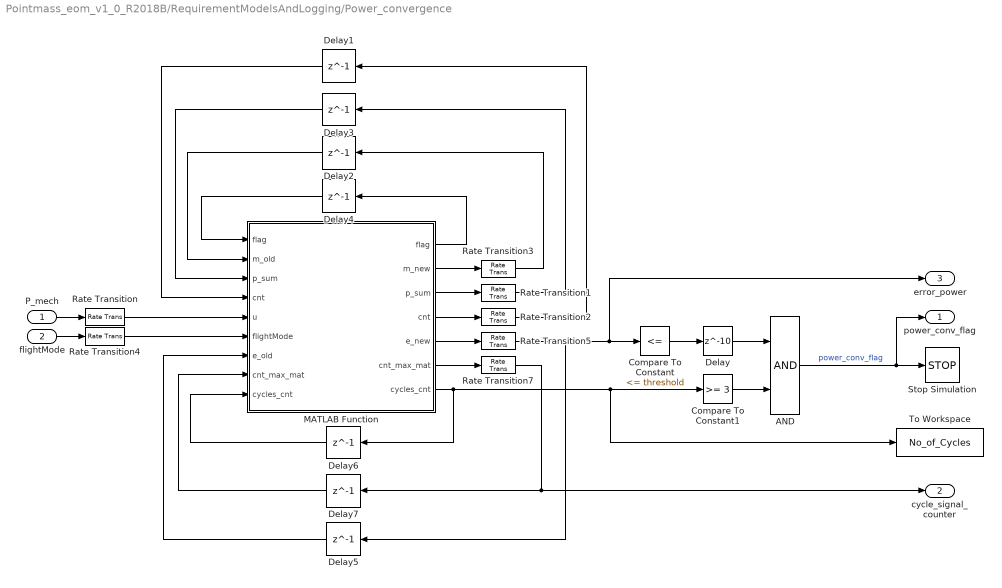
== system Pointmass_eom_v1_0_R2018B/RequirementModelsAndLogging/Power_convergence ==
  P_mech : Inport
  flightMode : Inport  Port=2
  AND : Logic  AllPortsSameDT=off  OutDataTypeStr=boolean
  Compare To Constant : simulink/Logic and Bit Operations/Compare To Constant  relop=<=  const=threshold  OutDataTypeStr=boolean
  Compare To Constant1 : simulink/Logic and Bit Operations/Compare To Constant  relop=>=  const=3  OutDataTypeStr=boolean
  Delay : Delay  DelayLength=10
  Delay{1..4,6..7} (6 alike) : Delay  DelayLength=1  InitialCondition=0
  Delay5 : Delay  DelayLength=1  InitialCondition=threshold+1000
  MATLAB Function : MATLAB Function  TreatAsAtomicUnit=on
  Rate Transition{,1..4,7} (6 alike) : RateTransition  OutPortSampleTime=sample_time
  Rate Transition5 : RateTransition  InitialCondition=1000  OutPortSampleTime=sample_time
  Stop Simulation : Stop
  To Workspace : ToWorkspace  VariableName=No_of_Cycles  SaveFormat=Timeseries  SampleTime=-1
      settings: MaxDataPoints=1
  power_conv_flag : Outport  VectorParamsAs1DForOutWhenUnconnected=off
  cycle_signal_counter : Outport  Port=2  VectorParamsAs1DForOutWhenUnconnected=off
  error_power : Outport  Port=3  VectorParamsAs1DForOutWhenUnconnected=off
  wires:
  MATLAB Function/4(cnt) -> Rate Transition2/1
  Delay1/1 -> MATLAB Function/4("cnt ")
  P_mech/1 -> Rate Transition/1
  Rate Transition/1 -> MATLAB Function/5(u)
  Rate Transition2/1 -> Delay1/1
  MATLAB Function/2(m_new) -> Rate Transition3/1
  Delay2/1 -> MATLAB Function/2(m_old)
  MATLAB Function/1(flag) -> Delay4/1
  Delay4/1 -> MATLAB Function/1("flag ")
  flightMode/1 -> Rate Transition4/1
  Delay3/1 -> MATLAB Function/3("p_sum ")
  Rate Transition1/1 -> Delay3/1
  MATLAB Function/3(p_sum) -> Rate Transition1/1
  Rate Transition4/1 -> MATLAB Function/6(flightMode)
  Rate Transition5/1 -> Compare To Constant/1, error_power/1, Delay5/1
  MATLAB Function/5(e_new) -> Rate Transition5/1
  Delay5/1 -> MATLAB Function/7(e_old)
  Compare To Constant/1 -> Delay/1
  AND/1 -> Stop Simulation/1, power_conv_flag/1  "power_conv_flag"
  Rate Transition7/1 -> Delay7/1, cycle_signal_counter/1
  MATLAB Function/6(cnt_max_mat) -> Rate Transition7/1
  Delay7/1 -> MATLAB Function/8("cnt_max_mat ")
  Rate Transition3/1 -> Delay2/1
  MATLAB Function/7(cycles_cnt) -> Compare To Constant1/1, To Workspace/1, Delay6/1
  Delay6/1 -> MATLAB Function/9("cycles_cnt ")
  Delay/1 -> AND/1
  Compare To Constant1/1 -> AND/2

== system Pointmass_eom_v1_0_R2018B/RequirementModelsAndLogging/Subsystem2 ==
  P_mech : Inport
  Constant7 : Constant
  Delay1 : Delay  DelayLength=1  SampleTime=0.1
  Delay3 : Delay  DelayLength=1  SampleTime=0.1
  Delay4 : Delay  DelayLength=1  InitialCondition=1  SampleTime=0.1
  Divide : Product  Inputs=*/
  Divide1 : Product  Inputs=*/
  Product : Product
  Rate Transition1 : RateTransition  OutPortSampleTime=0.1
  Rate Transition6 : RateTransition  OutPortSampleTime=0.1
  Sum : Sum  Inputs=|+-
  Sum1 : Sum  Inputs=|++
  Sum3 : Sum  Inputs=|++
  Sum4 : Sum  Inputs=|++
  To Workspace : ToWorkspace  Commented=on  VariableName=P_mech  SampleTime=log_sample_time
  mean_Pmech : Outport  VectorParamsAs1DForOutWhenUnconnected=off
  var_Pmech : Outport  Port=2  VectorParamsAs1DForOutWhenUnconnected=off
  wires:
  P_mech/1 -> Rate Transition6/1
  Delay4/1 -> Sum4/2
  Constant7/1 -> Rate Transition1/1
  Divide/1 -> mean_Pmech/1, Sum/2
  Rate Transition1/1 -> Sum4/1
  Sum3/1 -> Divide/1, Delay3/1
  Sum4/1 -> Divide1/2, Delay4/1, Divide/2
  Delay3/1 -> Sum3/2
  Sum/1 -> Product/2, Product/1
  Product/1 -> Sum1/1
  Delay1/1 -> Sum1/2
  Sum1/1 -> Divide1/1, Delay1/1
  Divide1/1 -> var_Pmech/1
  Rate Transition6/1 -> To Workspace/1, Sum/1, Sum3/1  "vel_w_W"

== system Pointmass_eom_v1_0_R2018B/AirborneSystem/AttitudeDynamics/SecondOrderReferenceModel_alpha_a ==
  y_cmd : Inport
  Constant : Constant  Value=omega0_max
  Discrete-Time Integrator : DiscreteIntegrator  SampleTime=-1  LimitOutput=on  UpperSaturationLimit=y_max  LowerSaturationLimit=y_min  ICPrevOutput=DiscIntNeverNeededParam  ICPrevScaledInput=DiscIntNeverNeededParam
  Discrete-Time Integrator1 : DiscreteIntegrator  SampleTime=-1  LimitOutput=on  UpperSaturationLimit=yd_max  LowerSaturationLimit=yd_min  ICPrevOutput=DiscIntNeverNeededParam  ICPrevScaledInput=DiscIntNeverNeededParam
  Gain2 : Gain  Gain=2*zeta0
  Product : Product  Inputs=3
  Product1 : Product
  Saturation : Saturate  UpperLimit=y_max  LowerLimit=y_min
  Saturation1 : Saturate  UpperLimit=y2d_max  LowerLimit=y2d_min
  Sum : Sum  Inputs=|+-
  Sum1 : Sum  Inputs=|+-
  y_ref : Outport  VectorParamsAs1DForOutWhenUnconnected=off
  wires:
  Discrete-Time Integrator/1 -> Sum1/2, y_ref/1
  Product/1 -> Sum/1
  y_cmd/1 -> Saturation/1
  Sum/1 -> Saturation1/1
  Gain2/1 -> Sum/2
  Sum1/1 -> Product/2
  Saturation1/1 -> Discrete-Time Integrator1/1
  Saturation/1 -> Sum1/1
  Discrete-Time Integrator1/1 -> Discrete-Time Integrator/1, Product1/1
  Product1/1 -> Gain2/1
  Constant/1 -> Product/1, Product/3, Product1/2

== system Pointmass_eom_v1_0_R2018B/AirborneSystem/AttitudeDynamics/SecondOrderReferenceModel_mu_a ==
  y_cmd : Inport
  Constant5 : Constant  Value=omega0_max
  Discrete-Time Integrator : DiscreteIntegrator  SampleTime=-1  LimitOutput=on  UpperSaturationLimit=y_max  LowerSaturationLimit=y_min  ICPrevOutput=DiscIntNeverNeededParam  ICPrevScaledInput=DiscIntNeverNeededParam
  Discrete-Time Integrator1 : DiscreteIntegrator  SampleTime=-1  LimitOutput=on  UpperSaturationLimit=yd_max  LowerSaturationLimit=yd_min  ICPrevOutput=DiscIntNeverNeededParam  ICPrevScaledInput=DiscIntNeverNeededParam
  Gain2 : Gain  Gain=2*zeta0
  Product : Product  Inputs=3
  Product1 : Product
  Saturation : Saturate  UpperLimit=y_max  LowerLimit=y_min
  Saturation1 : Saturate  UpperLimit=y2d_max  LowerLimit=y2d_min
  Sum : Sum  Inputs=|+-
  Sum1 : Sum  Inputs=|+-
  y_ref : Outport  VectorParamsAs1DForOutWhenUnconnected=off
  wires:
  Discrete-Time Integrator/1 -> Sum1/2, y_ref/1
  Product/1 -> Sum/1
  y_cmd/1 -> Saturation/1
  Sum/1 -> Saturation1/1
  Gain2/1 -> Sum/2
  Sum1/1 -> Product/2
  Saturation1/1 -> Discrete-Time Integrator1/1
  Saturation/1 -> Sum1/1
  Discrete-Time Integrator1/1 -> Discrete-Time Integrator/1, Product1/1
  Product1/1 -> Gain2/1
  Constant5/1 -> Product1/2, Product/3, Product/1

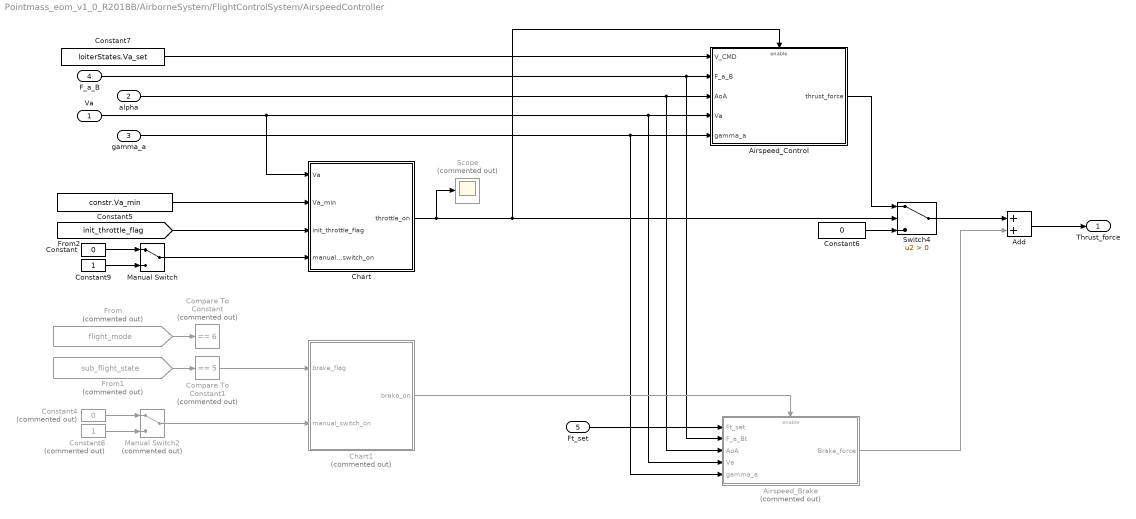
== system Pointmass_eom_v1_0_R2018B/AirborneSystem/FlightControlSystem/AirspeedController ==
  Va : Inport
  alpha : Inport  Port=2
  gamma_a : Inport  Port=3
  F_a_B : Inport  Port=4
  Ft_set : Inport  Port=5
  Add : Sum
  Airspeed_Brake : Subsystem  Commented=on
  Airspeed_Control : Subsystem
  Chart : Stateflow chart  TreatAsAtomicUnit=on
  Chart1 : Stateflow chart  Commented=on  TreatAsAtomicUnit=on
  Compare To Constant : simulink/Logic and Bit Operations/Compare To Constant  Commented=on  relop===  const=6  OutDataTypeStr=boolean
  Compare To Constant1 : simulink/Logic and Bit Operations/Compare To Constant  Commented=on  relop===  const=5  OutDataTypeStr=boolean
  Constant : Constant  Value=0
  Constant4 : Constant  Commented=on  Value=0
  Constant5 : Constant  Value=constr.Va_min
  Constant6 : Constant  Value=0
  Constant7 : Constant  Value=loiterStates.Va_set
  Constant8 : Constant  Commented=on
  Constant9 : Constant
  From : From  Commented=on  GotoTag=flight_mode  TagVisibility=global
  From1 : From  Commented=on  GotoTag=sub_flight_state  TagVisibility=global
  Manual Switch : ManualSwitch
  Manual Switch2 : ManualSwitch  Commented=on
  Scope : Scope  Commented=on
  Switch4 : Switch  Criteria=u2 > Threshold
  Thrust_force : Outport  VectorParamsAs1DForOutWhenUnconnected=off
  wires:
  Switch4/1 -> Add/1
  gamma_a/1 -> Airspeed_Control/5(gamma_a), Airspeed_Brake/5(gamma_a)
  F_a_B/1 -> Airspeed_Control/2(F_a_B), Airspeed_Brake/2(F_a_Bt)
  Constant6/1 -> Switch4/3
  Constant/1 -> Manual Switch/1
  Manual Switch/1 -> Chart/4(manual_switch_on)
  Constant7/1 -> Airspeed_Control/1(V_CMD)
  alpha/1 -> Airspeed_Control/3(AoA), Airspeed_Brake/3(AoA)
  [init_throttle_flag] -> Chart/3(init_throttle_flag)
  Constant9/1 -> Manual Switch/2
  Chart/1(throttle_on) -> Switch4/2, Airspeed_Control/Enable, Scope/1
  Va/1 -> Chart/1(Va), Airspeed_Control/4(Va), Airspeed_Brake/4(Va)
  Constant5/1 -> Chart/2(Va_min)
  Airspeed_Control/1(thrust_force) -> Switch4/1
  Chart1/1(brake_on) -> Airspeed_Brake/Enable
  Airspeed_Brake/1(Brake_force) -> Add/2
  Ft_set/1 -> Airspeed_Brake/1(Ft_set)
  Manual Switch2/1 -> Chart1/2(manual_switch_on)
  Compare To Constant1/1 -> Chart1/1(brake_flag)
  From1/1 -> Compare To Constant1/1
  From/1 -> Compare To Constant/1
  Add/1 -> Thrust_force/1
  Constant4/1 -> Manual Switch2/1
  Constant8/1 -> Manual Switch2/2
